simulink model "ABS_Regen_Straight"  (R2023a)
settings: Solver=ode45  StartTime=0  StopTime=15  FixedStep=0.002  RelTol=1e-3  AbsTol=1e-6
libraries: Solver_SF x1, cstblocks x1
settings Model: ExtModeTrigMode=oneshot  VariantFading=off  Creator=ywata  LastModifiedBy=USER
settings SolverCC: AutoScaleAbsTol=off  AlgebraicLoopSolver=TrustRegion
settings DataIOCC: SaveFormat=Array  SignalLoggingSaveFormat=ModelDataLogs  ReturnWorkspaceOutputs=off  SignalLoggingName=sigsOut
settings OptimizationCC: BlockReduction=off  BooleanDataType=off  ExpressionDepthLimit=2147483647  LifeSpan=inf
settings DebuggingCC: SaveWithParameterizedLinksMsg=none  UnderspecifiedInitializationDetection=Classic  MergeDetectMultiDrivingBlocksExec=none  SignalResolutionControl=TryResolveAllWithWarning  MultiTaskDSMMsg=warning  MultiTaskCondExecSysMsg=none  FcnCallInpInsideContextMsg=warning  UnconnectedInputMsg=warning  UnconnectedOutputMsg=warning  UnconnectedLineMsg=warning  StateNameClashWarn=warning  SFUnexpectedBacktrackingDiag=warning  SFNoUnconditionalDefaultTransitionDiag=warning  SFExecutionAtInitializationDiag=none  ArithmeticOperatorsInVariantConditions=warning
settings HardwareCC: ProdBitPerPointer=32  ProdBitPerSizeT=32  ProdBitPerPtrDiffT=32  ProdLargestAtomicFloat=None  ProdIntDivRoundTo=Undefined  ProdEndianess=Unspecified  ProdWordSize=32  ProdHWDeviceType=32-bit Generic  TargetUnknown=on
settings ModelReferenceCC: PropagateSignalLabelsOutOfModel=off
settings SFSimCC: SimUseLocalCustomCode=off  CustomCodeUndefinedFunction=UseInterfaceOnly
settings RTWCC: TemplateMakefile=grt_vc.tmf  RTWUseLocalCustomCode=off
settings CodeAppCC: StateflowObjectComments=on
settings GRTTargetCC: TargetFcnLib=ansi_tfl_tmw.mat  TargetLangStandard=C89/C90 (ANSI)  CombineOutputUpdateFcns=off  GRTInterface=on
settings ConfigComp: CovMetricSettings=dw  CovSaveCumulativeToWorkspaceVar=on  CovSaveSingleToWorkspaceVar=on  CovExternalEMLEnable=off

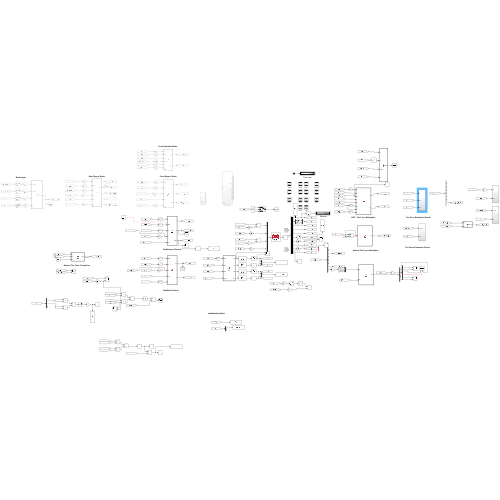
[thumbnail: Simulink's stored preview of the top-level diagram]
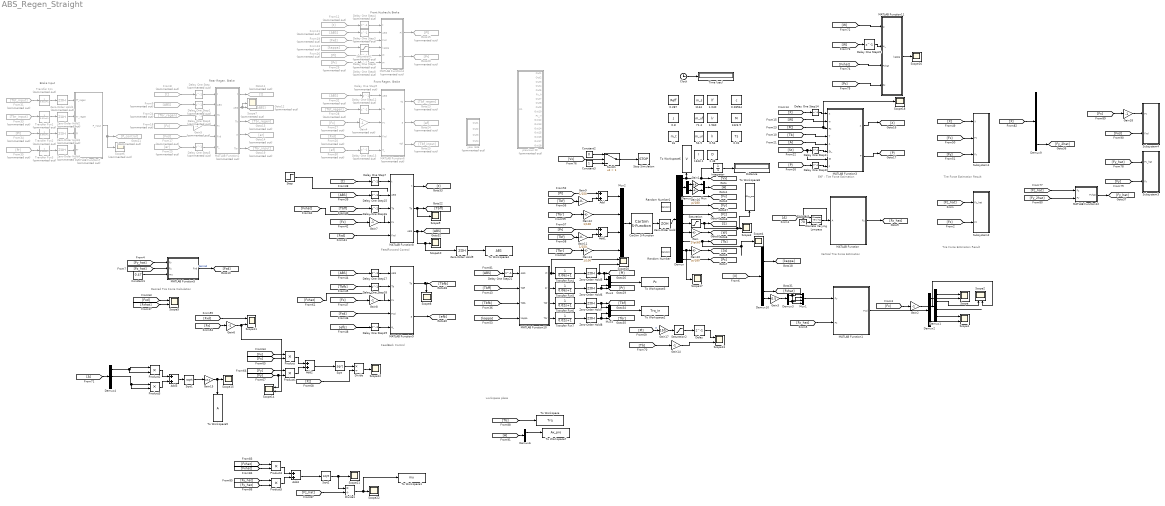
== system ABS_Regen_Straight ==
  note: workspace place
  note: Front Hydraulic Brake
  note: EKF : Tire Force Estimation
  note: Tire Force Estimation Result
  note: Vertical Tire Force Estimation
  note: Tire Force Estimation Result
  note: Rear Regen. Brake
  note: Desired Tire Force Calculation
  note: Front Regen. Brake
  note: Brake Input
  note: FeedForward Control
  note: FeedBack Control
  0.01 : DataStoreMemory  DataStoreName=Ts  WriteAfterWriteMsg=warning  InitialValue=0.01  ShowAdditionalParam=off  OutDataTypeStr=double
  0.287 : DataStoreMemory  DataStoreName=Reff  WriteAfterWriteMsg=warning  InitialValue=0.287  ShowAdditionalParam=off  OutDataTypeStr=double
  0.28944 : DataStoreMemory  DataStoreName=c  WriteAfterWriteMsg=warning  InitialValue=0.29844  ShowAdditionalParam=off  OutDataTypeStr=double
  0.54 : DataStoreMemory  DataStoreName=h  WriteAfterWriteMsg=warning  InitialValue=0.54  ShowAdditionalParam=off  OutDataTypeStr=double
  0.8 : DataStoreMemory  DataStoreName=J  WriteAfterWriteMsg=warning  InitialValue=0.8  ShowAdditionalParam=off  OutDataTypeStr=double
  1.040 : DataStoreMemory  DataStoreName=lf  WriteAfterWriteMsg=warning  InitialValue=1.040  ShowAdditionalParam=off  OutDataTypeStr=double
  1.48 : DataStoreMemory  DataStoreName=D  WriteAfterWriteMsg=warning  InitialValue=1.48  ShowAdditionalParam=off  OutDataTypeStr=double
  1.560 : DataStoreMemory  DataStoreName=lr  WriteAfterWriteMsg=warning  InitialValue=1.560  ShowAdditionalParam=off  OutDataTypeStr=double
  1134 : DataStoreMemory  DataStoreName=m_s  WriteAfterWriteMsg=warning  InitialValue=1134  ShowAdditionalParam=off  OutDataTypeStr=double
  1323.9 : DataStoreMemory  DataStoreName=M  WriteAfterWriteMsg=warning  InitialValue=1323.9  ShowAdditionalParam=off  OutDataTypeStr=double
  1343.1 : DataStoreMemory  DataStoreName=I  WriteAfterWriteMsg=warning  InitialValue=1343.1  ShowAdditionalParam=off  OutDataTypeStr=double
  16 : DataStoreMemory  DataStoreName=m_t  WriteAfterWriteMsg=warning  InitialValue=16  ShowAdditionalParam=off  OutDataTypeStr=double
  54.5 : DataStoreMemory  DataStoreName=m_ur  WriteAfterWriteMsg=warning  InitialValue=54.5  ShowAdditionalParam=off  OutDataTypeStr=double
  71.4 : DataStoreMemory  DataStoreName=m_uf  WriteAfterWriteMsg=warning  InitialValue=71.4  ShowAdditionalParam=off  OutDataTypeStr=double
  Add{,1..4} (5 alike) : Sum
  CarSim S-Function : Solver_SF/CarSim S-Function  Priority=1  SIMFILE=simfile.sim  Run_RTs=off  vs_state_ind=Run  StopMode_ind=Vehicle Model
  Clock : Clock
  Constant : Constant  Value=70  SampleTime=0.01
  Constant1 : Constant  Value=0.47
  Constant2 : Constant  Value=0
  Constant3 : Constant
  Delay : Delay  DelayLength=1
  Delay One Step : Delay  Commented=on  DelayLength=1  InitialCondition=-0.01
  Delay One Step{1,3,5..6,8..9,13} (7 alike) : Delay  Commented=on  DelayLength=1  InitialCondition=0
  Delay One Step10 : Delay  DelayLength=1  InitialCondition=diag([67.655 67.655 67.655 67.655 10 0 0 0 0 0 0 0 0 0 0 0])
  Delay One Step11 : Delay  DelayLength=1  InitialCondition=[0 0]'
  Delay One Step12 : Delay  Commented=on  DelayLength=1  InitialCondition=[0 0 0 0]'
  Delay One Step14 : Delay  DelayLength=1  InitialCondition=[67.655 67.655 67.655 67.655 10 0 0 0 0 0 0 0 0 0 0 0]'
  Delay One Step15 : Delay  DelayLength=1  InitialCondition=0
  Delay One Step16 : Delay  DelayLength=1  InitialCondition=[0 0 0 0]'
  Delay One Step17 : Delay  DelayLength=1  InitialCondition=0
  Delay One Step18 : Delay  DelayLength=1  InitialCondition=[0 0 0 0]'
  Delay One Step19 : Delay  DelayLength=1  InitialCondition=[0 0 0 0]'
  Delay One Step2 : Delay  Commented=on  DelayLength=1  InitialCondition=[0 0 0 0]'
  Delay One Step20 : Delay  DelayLength=1  InitialCondition=[67.655,67.655,67.655,67.655]'
  Delay One Step21 : Delay  DelayLength=1  InitialCondition=0
  Delay One Step4 : Delay  Commented=on  DelayLength=1  InitialCondition=-0.01
  Delay One Step7 : Delay  DelayLength=1  InitialCondition=-0.01
  Demux : Demux  Outputs=[1 3 4 4 4 4 4 4 2 2]
  Demux1 : Demux
  Demux10 : Demux  Outputs=[4 1 2 1 2 4 2]
  Demux2 : Demux
  Demux3 : Demux  Outputs=2
  Demux4 : Demux  Outputs=3
  Demux5 : Demux  Outputs=[2 1]
  Demux6 : Demux  Outputs=3
  Demux9 : Demux  Outputs=[4 1 2 1 2 4 2]
  Discrete Varying Lowpass : cstblocks/Linear Parameter Varying/Discrete Varying Lowpass  N=1  w0=0  Ts=0.01
  Distance : Display
      settings: Format=bank  Decimation=100
  Divide : Product  Inputs=*/
  Divide1 : Product  Inputs=*/
  From{1,21,71,91} (4 alike) : From
  From11 : From  Commented=on  GotoTag=ABS
  From12 : From  Commented=on  GotoTag=t
  From13 : From  Commented=on  GotoTag=kappa
  From17 : From  Commented=on  GotoTag=Fxd
  From18 : From  Commented=on  GotoTag=Fx
  From19 : From  Commented=on  GotoTag=Fxd
  From20 : From  Commented=on  GotoTag=Fxd
  From24 : From  Commented=on  GotoTag=Tbr_regen
  From25 : From  Commented=on  GotoTag=er
  From26 : From  Commented=on  GotoTag=Pl
  From27 : From  Commented=on  GotoTag=Fx
  From28 : From  Commented=on  GotoTag=Tbf_regen
  From29 : From  Commented=on  GotoTag=Pr
  From30 : From  Commented=on  GotoTag=ef
  From31 : From  Commented=on  GotoTag=Tbf_input
  From32 : From  Commented=on  GotoTag=ABS
  From33 : From  Commented=on  GotoTag=Tbr_input
  From34 : From  Commented=on  GotoTag=Pl
  From35 : From  Commented=on  GotoTag=Pr
  From8 : From  Commented=on  GotoTag=t
  From9 : From  Commented=on  GotoTag=ABS
  Gain : Gain  Gain=2*pi/60
  Gain1 : Gain  Gain=9.8
  Gain10 : Gain  Gain=pi/180
  Gain11 : Gain  Gain=1/150
  Gain12 : Gain  Gain=1/100
  Gain13 : Gain  Gain=1/100
  Gain{2,6..8,14,18} (6 alike) : Gain  Gain=-1
  Gain15 : Gain  Gain=1/9.8
  Gain16 : Gain  Gain=pi/180
  Gain17 : Gain  Gain=150
  Gain3 : Gain  Gain=0.5
  Gain4 : Gain  Commented=on  Gain=-1
  Gain5 : Gain  Commented=on  Gain=-1
  Gain9 : Gain  Gain=1/150
  Goto1 : Goto
  Goto11 : Goto  Commented=on  GotoTag=t
  Goto12 : Goto  Commented=on  GotoTag=ABS
  Goto13 : Goto  Commented=on  GotoTag=Tbr_regen
  Goto14 : Goto  Commented=on  GotoTag=er
  Goto15 : Goto  Commented=on  GotoTag=Pl
  Goto19 : Goto  Commented=on  GotoTag=Tbr_input
  Goto20 : Goto  Commented=on  GotoTag=Pr
  Goto21 : Goto  Commented=on  GotoTag=P_control
  Goto23 : Goto  Commented=on  GotoTag=Tbf_regen
  Goto24 : Goto  Commented=on  GotoTag=ef
  Goto25 : Goto  Commented=on  GotoTag=Tbf_input
  Integrator : Integrator
  MATLAB Function : MATLAB Function  TreatAsAtomicUnit=on
  MATLAB Function1 : MATLAB Function  TreatAsAtomicUnit=on
  MATLAB Function10 : MATLAB Function  TreatAsAtomicUnit=on
  MATLAB Function11 : MATLAB Function  TreatAsAtomicUnit=on
  MATLAB Function12 : MATLAB Function  TreatAsAtomicUnit=on
  MATLAB Function2 : MATLAB Function  Commented=on  TreatAsAtomicUnit=on
  MATLAB Function3 : MATLAB Function  TreatAsAtomicUnit=on
  MATLAB Function4 : MATLAB Function  Commented=on  TreatAsAtomicUnit=on
  MATLAB Function5 : MATLAB Function  TreatAsAtomicUnit=on
  MATLAB Function6 : MATLAB Function  Commented=on  TreatAsAtomicUnit=on
  MATLAB Function7 : MATLAB Function  Commented=on  TreatAsAtomicUnit=on
  MATLAB Function8 : MATLAB Function  TreatAsAtomicUnit=on
  MATLAB Function9 : MATLAB Function  TreatAsAtomicUnit=on
  Mux : Mux  Inputs=2
  Mux1 : Mux
  Mux2 : Mux
  Mux3 : Mux  Inputs=2
  Mux4 : Mux  Inputs=2
  Product{,1..5} (6 alike) : Product
  Random Number : RandomNumber  Variance=0.01^2  SampleTime=0.01
  Random Number1 : RandomNumber  Variance=0.01  SampleTime=0.01
  Saturation : Saturate  UpperLimit=1  LowerLimit=-1
  Saturation1 : Saturate  Commented=on  UpperLimit=200  LowerLimit=100
  Saturation2 : Saturate  UpperLimit=1000  LowerLimit=0
  Scope{,1..2,5,11,13..14,20} (8 alike) : Scope  NumInputPorts=2
  Scope{3..4,8..10,12,15..18,21..22} (12 alike) : Scope
  Scope6 : Scope  Commented=on
  Scope7 : Scope  Commented=on
  Sqrt : Sqrt
  Sqrt1 : Sqrt
  Sqrt2 : Sqrt
  Step : Step  Time=5.34  SampleTime=0.01
  Stop Simulation : Stop
  Subsystem1 : Subsystem
  Subsystem2 : Subsystem
  Subsystem3 : Subsystem
  Subsystem4 : Subsystem
  Switch : Switch  Criteria=u2 > Threshold  Threshold=1  SaturateOnIntegerOverflow=off  InputSameDT=off
  Time (sec) : Display
      settings: Format=bank  Decimation=100
  To Workspace : ToWorkspace  VariableName=Trq  SaveFormat=Timeseries  SampleTime=-1
  To Workspace1 : ToWorkspace  VariableName=mu  SaveFormat=Timeseries  SampleTime=-1
  To Workspace2 : ToWorkspace  VariableName=Trq_in  SaveFormat=Timeseries  SampleTime=-1
  To Workspace3 : ToWorkspace  VariableName=Pc  SaveFormat=Timeseries  SampleTime=-1
  To Workspace4 : ToWorkspace  VariableName=ABS  SaveFormat=Timeseries  SampleTime=-1
  To Workspace5 : ToWorkspace  VariableName=A  SaveFormat=Timeseries  SampleTime=-1
  To Workspace6 : ToWorkspace  VariableName=V  SaveFormat=Timeseries  SampleTime=-1
  To Workspace7 : ToWorkspace  VariableName=Ax_pro  SaveFormat=Timeseries  SampleTime=-1
  To Workspace8 : ToWorkspace  VariableName=Slip_pro  SaveFormat=Timeseries  SampleTime=-1
  Transfer Fcn : TransferFcn  Commented=on  Denominator=[0.02 1]
  Transfer Fcn1 : TransferFcn  Commented=on  Denominator=[0.02 1]
  Transfer Fcn2 : TransferFcn  Commented=on  Denominator=[0.06 1]
  Transfer Fcn3 : TransferFcn  Commented=on  Denominator=[0.06 1]
  Transfer Fcn4 : TransferFcn  Denominator=[0.06 1]
  Transfer Fcn5 : TransferFcn  Denominator=[0.06 1]
  Transfer Fcn6 : TransferFcn  Denominator=[0.02 1]
  Transfer Fcn7 : TransferFcn  Denominator=[0.02 1]
  Zero-Order Hold{,5..9} (6 alike) : ZeroOrderHold  SampleTime=0.01
  Zero-Order Hold{1..4} (4 alike) : ZeroOrderHold  Commented=on  SampleTime=0.01
  previous KF : Subsystem  Commented=on
  yaw rate : Subsystem  Commented=on
  wires:
  CarSim S-Function/1 -> Zero-Order Hold/1
  Clock/1 -> Time (sec)/1
  Demux/1 -> Integrator/1, [Vx], To Workspace6/1
  Demux/3 -> [Fx]
  Zero-Order Hold/1 -> Demux/1
  Saturation/1 -> To Workspace8/1, Scope3/1, [S]
  Gain/1 -> [W]
  Demux/2 -> Demux5/1
  Demux5/1 -> Gain1/1
  Mux/1 -> Goto1/1
  Demux5/2 -> Gain16/1
  Gain1/1 -> Mux/1
  Demux/10 -> [Pc]
  Demux/9 -> Scope17/1, Gain10/1
  Demux/8 -> Scope4/1, [Tb]
  Demux/7 -> Gain/1
  Demux/6 -> Saturation/1
  Demux/5 -> [Fz]
  Demux/4 -> [Fy]
  Gain16/1 -> Mux/2
  Delay One Step11/1 -> MATLAB Function3/6(St_)
  From21/1 -> MATLAB Function3/5(A)
  [P] -> Delay One Step10/1
  [Tb] -> MATLAB Function3/4(T)
  [W] -> MATLAB Function3/2(w)
  [X] -> Delay One Step14/1
  [St] -> MATLAB Function3/7(St), Delay One Step11/1
  MATLAB Function3/2(P) -> [P]
  Delay One Step10/1 -> MATLAB Function3/8("P ")
  MATLAB Function3/1(X) -> [X]
  [Pc] -> Scope18/1, MATLAB Function3/3(Pc)
  Delay One Step14/1 -> MATLAB Function3/1("X ")
  Gain10/1 -> [St]
  [X] -> Subsystem1/1(X)
  [Fx] -> Subsystem1/2(Fx)
  [Fy] -> Subsystem1/3(Fy)
  From1/1 -> MATLAB Function/1(A), Discrete Varying Lowpass/1
  MATLAB Function/1(Fz) -> [Fz_hat]
  [Fz_hat] -> Subsystem2/1(Fz_hat)
  [Fz] -> Subsystem2/2(Fz)
  Constant/1 -> Discrete Varying Lowpass/2
  Discrete Varying Lowpass/1 -> ?
  [Fz_hat] -> MATLAB Function1/2(Fz)
  MATLAB Function1/1(Fxd) -> Demux2/1
  [Fx] -> Gain2/1
  Gain2/1 -> Demux1/1
  Demux1/1 -> Scope/1
  Demux2/1 -> Scope/2
  Demux1/4 -> Scope1/1
  Demux2/4 -> Scope1/2
  [X] -> Demux10/1
  Demux10/7 -> Gain3/1
  Gain3/1 -> Demux3/1
  Demux3/1 -> Mux1/3, Mux1/1
  Mux1/1 -> MATLAB Function1/1(Fy)
  Demux3/2 -> Mux1/4, Mux1/2
  Demux1/2 -> Scope2/1
  Demux1/3 -> ?
  MATLAB Function2/1(t) -> Goto11/1
  MATLAB Function2/2(ABS) -> Scope7/1, Goto12/1
  [Fy_hat] -> MATLAB Function5/1(Fy)
  [Fz_hat] -> MATLAB Function5/2(Fz)
  MATLAB Function5/1(Fxd) -> [Fxd]  "desired"
  From8/1 -> Delay One Step/1
  Delay One Step/1 -> MATLAB Function2/1("t ")
  From9/1 -> Delay One Step1/1
  Delay One Step1/1 -> MATLAB Function2/2("ABS ")
  From11/1 -> Delay One Step3/1
  Delay One Step3/1 -> MATLAB Function4/2(ABS)
  From12/1 -> Delay One Step4/1
  Delay One Step4/1 -> MATLAB Function4/1(t)
  From17/1 -> MATLAB Function2/5(Fxd)
  From18/1 -> Gain5/1
  Gain5/1 -> MATLAB Function2/4(Fx)
  From19/1 -> MATLAB Function4/3(Fxd)
  MATLAB Function2/3(Tb) -> Goto13/1
  From24/1 -> Delay One Step2/1
  Delay One Step2/1 -> MATLAB Function2/3("Tb ")
  MATLAB Function2/4(e) -> Goto14/1
  From25/1 -> Delay One Step5/1
  Delay One Step5/1 -> MATLAB Function2/6(e_)
  Demux10/2 -> [kappa]
  From13/1 -> Saturation1/1
  MATLAB Function2/5(Tbr) -> Goto19/1
  MATLAB Function4/1(Pl) -> Goto15/1
  MATLAB Function4/2(Pr) -> Goto20/1
  From26/1 -> Delay One Step6/1
  Delay One Step6/1 -> MATLAB Function4/5("Pl ")
  Delay One Step8/1 -> MATLAB Function4/6("Pr ")
  From29/1 -> Delay One Step8/1
  Saturation1/1 -> MATLAB Function4/4(kappa)
  From30/1 -> Delay One Step13/1
  From28/1 -> Delay One Step12/1
  Delay One Step12/1 -> MATLAB Function6/2("Tb ")
  Delay One Step13/1 -> MATLAB Function6/5(e_)
  MATLAB Function6/1(Tb) -> Goto23/1
  From27/1 -> Gain4/1
  Delay One Step9/1 -> MATLAB Function6/1(ABS)
  MATLAB Function6/2(e) -> Goto24/1
  Gain4/1 -> MATLAB Function6/3(Fx)
  MATLAB Function6/3(Tbf) -> Goto25/1
  From32/1 -> Delay One Step9/1
  From20/1 -> MATLAB Function6/4(Fxd)
  From31/1 -> Transfer Fcn/1
  From33/1 -> Transfer Fcn1/1
  From34/1 -> Transfer Fcn2/1
  From35/1 -> Transfer Fcn3/1
  MATLAB Function7/1(P_input) -> Scope6/1, Goto21/1
  Transfer Fcn/1 -> Zero-Order Hold1/1
  Transfer Fcn1/1 -> Zero-Order Hold2/1
  Transfer Fcn2/1 -> Zero-Order Hold3/1
  Transfer Fcn3/1 -> Zero-Order Hold4/1
  Zero-Order Hold1/1 -> MATLAB Function7/1(Tf_regen)
  Zero-Order Hold2/1 -> MATLAB Function7/2(Tr_regen)
  Zero-Order Hold3/1 -> MATLAB Function7/3(Pl)
  Zero-Order Hold4/1 -> MATLAB Function7/4(Pr)
  Constant1/1 -> MATLAB Function5/3(mu)
  [ABS] -> Delay One Step15/1
  Delay One Step7/1 -> MATLAB Function8/1("t ")
  [t] -> Delay One Step7/1
  Delay One Step15/1 -> MATLAB Function8/2("ABS ")
  MATLAB Function8/2(Tb) -> Scope9/1, [Tbff]
  [Tbff] -> Delay One Step16/1
  Delay One Step16/1 -> MATLAB Function8/3("Tb ")
  Gain7/1 -> ?
  [Fxd] -> MATLAB Function8/5(Fxd)
  [Fx] -> Gain7/1
  [Fxd] -> MATLAB Function9/4(Fxd)
  Delay One Step18/1 -> MATLAB Function9/2("Tb ")
  [Fx] -> Gain8/1
  [Tbfb] -> Delay One Step18/1
  Gain8/1 -> ?
  Delay One Step17/1 -> MATLAB Function9/1(ABS)
  [ABS] -> Delay One Step17/1
  MATLAB Function9/2(e) -> [efb]
  MATLAB Function9/1(Tb) -> Scope8/1, [Tbfb]
  [efb] -> Delay One Step19/1
  Delay One Step19/1 -> MATLAB Function9/5(e_)
  Demux10/6 -> [Fxhat]
  MATLAB Function8/3(ABS) -> Zero-Order Hold9/1, Scope10/1, [ABS]
  MATLAB Function8/1(t) -> [t]
  [Fxd] -> Scope11/1
  [Fx] -> Gain6/1
  [Tbfb] -> MATLAB Function10/3(Tbfb)
  [Tbff] -> MATLAB Function10/2(Tbff)
  [kappa] -> MATLAB Function10/4(kappa)
  MATLAB Function10/1(Pl) -> Scope20/1, Transfer Fcn4/1
  Add/1 -> Mux2/1
  [Pl] -> Add/1
  [Tbf] -> Gain9/1
  Gain9/1 -> Add/2
  [Tbf] -> Gain11/1
  Add1/1 -> Mux2/3
  [Pr] -> Add1/1
  Gain11/1 -> Add1/2
  MATLAB Function10/2(Pr) -> Transfer Fcn5/1
  MATLAB Function10/3(Tbf) -> Transfer Fcn6/1
  MATLAB Function10/4(Tbr) -> Transfer Fcn7/1
  [Tbr] -> Gain12/1
  Gain12/1 -> Mux2/2
  Gain13/1 -> Mux2/4
  [Tbr] -> Gain13/1
  [Fxhat] -> MATLAB Function9/3(Fx)
  [Fxhat] -> MATLAB Function8/4(Fx)
  [Fxd] -> Scope5/1
  Gain6/1 -> Scope11/2, Scope14/2
  [Fxhat] -> Scope5/2
  Transfer Fcn4/1 -> Zero-Order Hold5/1
  Transfer Fcn5/1 -> Zero-Order Hold6/1
  Transfer Fcn6/1 -> Zero-Order Hold7/1
  Transfer Fcn7/1 -> Zero-Order Hold8/1
  Zero-Order Hold5/1 -> Scope20/2, Mux3/1, [Pl]
  Zero-Order Hold6/1 -> Mux3/2, [Pr]
  Zero-Order Hold7/1 -> Mux4/1, [Tbf]
  Zero-Order Hold8/1 -> Mux4/2, [Tbr]
  [Fx] -> Product/1
  [Fx] -> Product/2
  [Fy] -> Scope14/1, Product1/2
  [Fy] -> Product1/1
  Product/1 -> Add2/1
  Product1/1 -> Add2/2
  Add2/1 -> Sqrt/1
  Sqrt/1 -> Divide/1
  [Fz] -> Divide/2
  Divide/1 -> Scope12/1
  [Pl] -> Gain17/1  "in"
  [Tb] -> Gain14/1
  Gain14/1 -> Scope13/2
  Saturation2/1 -> Delay/1
  Delay/1 -> Scope13/1
  From71/1 -> Demux4/1
  Product3/1 -> Add3/2
  Product2/1 -> Add3/1
  Add3/1 -> Sqrt1/1
  Demux4/1 -> Product2/2, Product2/1
  Demux4/2 -> Product3/2, Product3/1
  Sqrt1/1 -> Gain15/1
  Gain15/1 -> To Workspace5/1, Scope15/1
  Demux2/2 -> Scope2/2
  [W] -> MATLAB Function11/1(w)
  [W] -> Delay One Step20/1
  Delay One Step20/1 -> MATLAB Function11/2(w_)
  [Pc] -> MATLAB Function11/4(Pc)
  [Fxhat] -> MATLAB Function11/3(Fxhat)
  MATLAB Function11/1(kappa) -> Scope16/1
  [Vx] -> Switch/2
  Constant2/1 -> Switch/1
  Constant3/1 -> Switch/3
  Switch/1 -> Stop Simulation/1
  [X] -> Demux9/1
  Demux9/7 -> [Fy_2hat]
  [Fz_hat] -> MATLAB Function12/1(Fz)
  [Fy_2hat] -> MATLAB Function12/2(Fy)
  MATLAB Function12/1(Fyhat) -> [Fy_hat]
  [Fy] -> Subsystem3/2(Fy)
  [Fy_hat] -> Subsystem3/1(Fy_hat)
  Gain17/1 -> Saturation2/1
  [ABS] -> Delay One Step21/1
  Delay One Step21/1 -> MATLAB Function10/1(ABS)
  Product4/1 -> Add4/1
  [Fy_hat] -> Product5/2
  [Fy_hat] -> Product5/1
  [Fxhat] -> Product4/2
  Add4/1 -> Sqrt2/1
  [Fxhat] -> Product4/1
  Product5/1 -> Add4/2
  Sqrt2/1 -> Divide1/1, Scope21/1
  [Fz_hat] -> Divide1/2
  Divide1/1 -> To Workspace1/1, Scope22/1
  [Tb] -> To Workspace/1
  Mux3/1 -> To Workspace3/1
  Mux4/1 -> To Workspace2/1
  Zero-Order Hold9/1 -> To Workspace4/1
  [Fxd] -> Subsystem4/2(Fxd)
  [Fx] -> Gain18/1
  From91/1 -> Demux6/1
  Demux6/1 -> To Workspace7/1
  Integrator/1 -> Distance/1
  Gain18/1 -> Subsystem4/1(Fx)
  Step/1 -> ?
  Mux2/1 -> CarSim S-Function/1

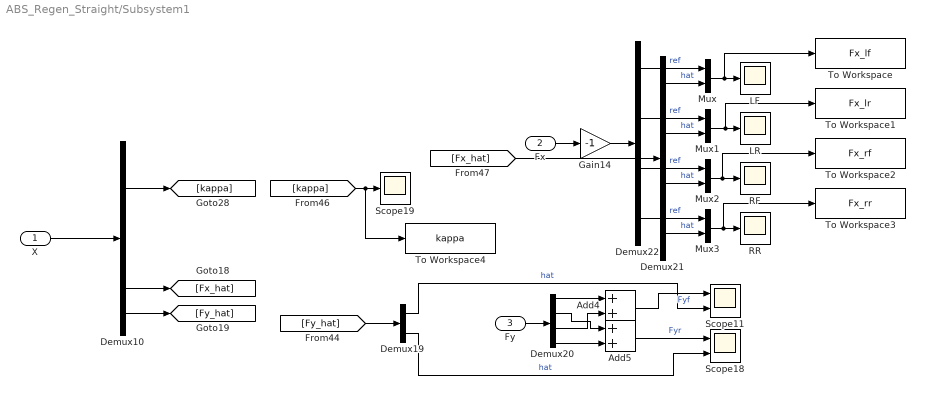
== system ABS_Regen_Straight/Subsystem1 ==
  X : Inport
  Fx : Inport  Port=2
  Fy : Inport  Port=3
  Add4 : Sum
  Add5 : Sum
  Demux10 : Demux  Outputs=[4 1 2 1 2 4 2]
  Demux19 : Demux  Outputs=2
  Demux20 : Demux
  Demux21 : Demux
  Demux22 : Demux
  Gain14 : Gain  Gain=-1
  LF : Scope
  LR : Scope
  Mux{,1..3} (4 alike) : Mux  Inputs=2
  RF : Scope
  RR : Scope
  Scope11 : Scope  NumInputPorts=2
  Scope18 : Scope  NumInputPorts=2
  Scope19 : Scope
  To Workspace : ToWorkspace  VariableName=Fx_lf  SaveFormat=Timeseries  SampleTime=-1
  To Workspace1 : ToWorkspace  VariableName=Fx_lr  SaveFormat=Timeseries  SampleTime=-1
  To Workspace2 : ToWorkspace  VariableName=Fx_rf  SaveFormat=Timeseries  SampleTime=-1
  To Workspace3 : ToWorkspace  VariableName=Fx_rr  SaveFormat=Timeseries  SampleTime=-1
  To Workspace4 : ToWorkspace  VariableName=kappa  SaveFormat=Timeseries  SampleTime=-1
  wires:
  Demux21/3 -> Mux2/2  "hat"
  [Fx_hat] -> Demux21/1
  Add5/1 -> Scope18/1  "Fyr"
  [Fy_hat] -> Demux19/1
  Demux21/4 -> Mux3/2  "hat"
  Fx/1 -> Gain14/1
  Gain14/1 -> Demux22/1
  Demux22/4 -> Mux3/1  "ref"
  Demux20/1 -> Add4/1
  Demux10/2 -> [kappa]
  Demux19/1 -> Scope11/2  "hat"
  Demux19/2 -> Scope18/2  "hat"
  Demux21/1 -> Mux/2  "hat"
  Demux20/2 -> Add5/1
  Demux22/3 -> Mux2/1  "ref"
  Demux20/4 -> Add5/2
  Demux20/3 -> Add4/2
  Demux10/7 -> [Fy_hat]
  Fy/1 -> Demux20/1
  Demux22/2 -> Mux1/1  "ref"
  Demux21/2 -> Mux1/2  "hat"
  X/1 -> Demux10/1
  Add4/1 -> Scope11/1  "Fyf"
  Demux10/6 -> [Fx_hat]
  [kappa] -> To Workspace4/1, Scope19/1
  Demux22/1 -> Mux/1  "ref"
  Mux/1 -> To Workspace/1, LF/1
  Mux1/1 -> To Workspace1/1, LR/1
  Mux2/1 -> To Workspace2/1, RF/1
  Mux3/1 -> To Workspace3/1, RR/1

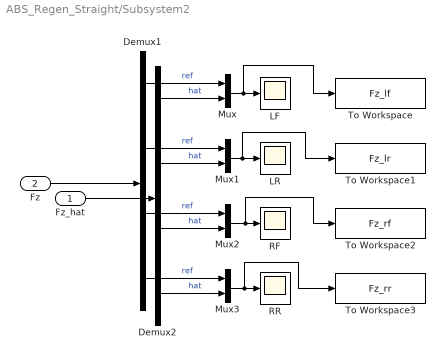
== system ABS_Regen_Straight/Subsystem2 ==
  Fz_hat : Inport
  Fz : Inport  Port=2
  Demux1 : Demux
  Demux2 : Demux
  LF : Scope
  LR : Scope
  Mux{,1..3} (4 alike) : Mux  Inputs=2
  RF : Scope
  RR : Scope
  To Workspace : ToWorkspace  VariableName=Fz_lf  SaveFormat=Timeseries  SampleTime=-1
  To Workspace1 : ToWorkspace  VariableName=Fz_lr  SaveFormat=Timeseries  SampleTime=-1
  To Workspace2 : ToWorkspace  VariableName=Fz_rf  SaveFormat=Timeseries  SampleTime=-1
  To Workspace3 : ToWorkspace  VariableName=Fz_rr  SaveFormat=Timeseries  SampleTime=-1
  wires:
  Fz_hat/1 -> Demux2/1
  Fz/1 -> Demux1/1
  Demux1/1 -> Mux/1  "ref"
  Demux2/1 -> Mux/2  "hat"
  Demux2/2 -> Mux1/2  "hat"
  Demux1/2 -> Mux1/1  "ref"
  Demux1/3 -> Mux2/1  "ref"
  Demux2/3 -> Mux2/2  "hat"
  Demux1/4 -> Mux3/1  "ref"
  Demux2/4 -> Mux3/2  "hat"
  Mux/1 -> To Workspace/1, LF/1
  Mux1/1 -> To Workspace1/1, LR/1
  Mux2/1 -> To Workspace2/1, RF/1
  Mux3/1 -> To Workspace3/1, RR/1

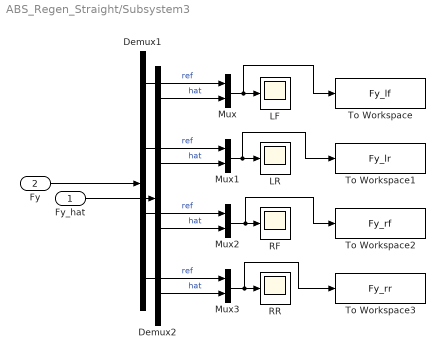
== system ABS_Regen_Straight/Subsystem3 ==
  Fy_hat : Inport
  Fy : Inport  Port=2
  Demux1 : Demux
  Demux2 : Demux
  LF : Scope
  LR : Scope
  Mux{,1..3} (4 alike) : Mux  Inputs=2
  RF : Scope
  RR : Scope
  To Workspace : ToWorkspace  VariableName=Fy_lf  SaveFormat=Timeseries  SampleTime=-1
  To Workspace1 : ToWorkspace  VariableName=Fy_lr  SaveFormat=Timeseries  SampleTime=-1
  To Workspace2 : ToWorkspace  VariableName=Fy_rf  SaveFormat=Timeseries  SampleTime=-1
  To Workspace3 : ToWorkspace  VariableName=Fy_rr  SaveFormat=Timeseries  SampleTime=-1
  wires:
  Fy_hat/1 -> Demux2/1
  Fy/1 -> Demux1/1
  Demux1/1 -> Mux/1  "ref"
  Demux2/1 -> Mux/2  "hat"
  Demux2/2 -> Mux1/2  "hat"
  Demux1/2 -> Mux1/1  "ref"
  Demux1/3 -> Mux2/1  "ref"
  Demux2/3 -> Mux2/2  "hat"
  Demux1/4 -> Mux3/1  "ref"
  Demux2/4 -> Mux3/2  "hat"
  Mux/1 -> To Workspace/1, LF/1
  Mux1/1 -> To Workspace1/1, LR/1
  Mux2/1 -> To Workspace2/1, RF/1
  Mux3/1 -> To Workspace3/1, RR/1

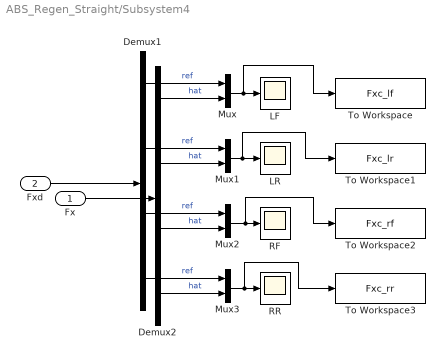
== system ABS_Regen_Straight/Subsystem4 ==
  Fx : Inport
  Fxd : Inport  Port=2
  Demux1 : Demux
  Demux2 : Demux
  LF : Scope
  LR : Scope
  Mux{,1..3} (4 alike) : Mux  Inputs=2
  RF : Scope
  RR : Scope
  To Workspace : ToWorkspace  VariableName=Fxc_lf  SaveFormat=Timeseries  SampleTime=-1
  To Workspace1 : ToWorkspace  VariableName=Fxc_lr  SaveFormat=Timeseries  SampleTime=-1
  To Workspace2 : ToWorkspace  VariableName=Fxc_rf  SaveFormat=Timeseries  SampleTime=-1
  To Workspace3 : ToWorkspace  VariableName=Fxc_rr  SaveFormat=Timeseries  SampleTime=-1
  wires:
  Fx/1 -> Demux2/1
  Fxd/1 -> Demux1/1
  Demux1/1 -> Mux/1  "ref"
  Demux2/1 -> Mux/2  "hat"
  Demux2/2 -> Mux1/2  "hat"
  Demux1/2 -> Mux1/1  "ref"
  Demux1/3 -> Mux2/1  "ref"
  Demux2/3 -> Mux2/2  "hat"
  Demux1/4 -> Mux3/1  "ref"
  Demux2/4 -> Mux3/2  "hat"
  Mux/1 -> To Workspace/1, LF/1
  Mux1/1 -> To Workspace1/1, LR/1
  Mux2/1 -> To Workspace2/1, RF/1
  Mux3/1 -> To Workspace3/1, RR/1

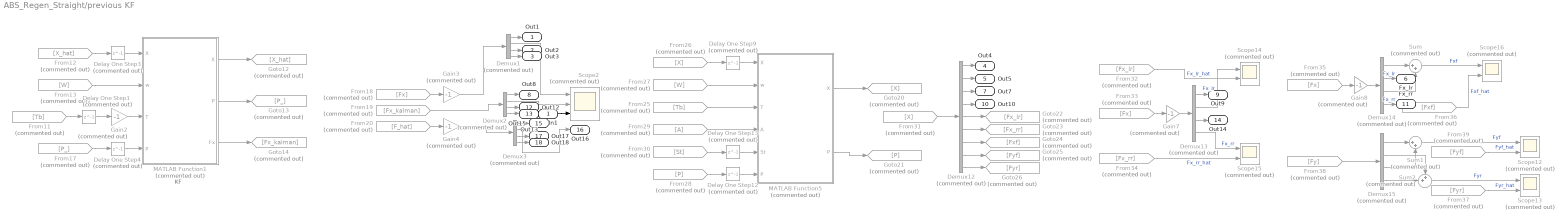
== system ABS_Regen_Straight/previous KF ==
  note: KF
  In1 : Inport
  Delay One Step1 : Delay  Commented=on  DelayLength=1  InitialCondition=zeros(4,1)
  Delay One Step12 : Delay  Commented=on  DelayLength=1  InitialCondition=diag([67.655 67.655 0 0 0 0 0 0 0])
  Delay One Step13 : Delay  Commented=on  DelayLength=1  InitialCondition=[0 0]'
  Delay One Step3 : Delay  Commented=on  DelayLength=1  InitialCondition=[67.655 67.655 67.655 67.655; 0 0 0 0]
  Delay One Step4 : Delay  Commented=on  DelayLength=1  InitialCondition=10*ones(2,8)
  Delay One Step9 : Delay  Commented=on  DelayLength=1  InitialCondition=[67.655 67.655 0 0 0 0 0 0 0]'
  Demux{1..3,13..15} (6 alike) : Demux  Commented=on
  Demux12 : Demux  Commented=on  Outputs=9
  From11 : From  Commented=on  GotoTag=Tb
  From12 : From  Commented=on  GotoTag=X_hat
  From13 : From  Commented=on  GotoTag=W
  From17 : From  Commented=on  GotoTag=P_
  From18 : From  Commented=on  GotoTag=Fx
  From19 : From  Commented=on  GotoTag=Fx_kalman
  From20 : From  Commented=on  GotoTag=F_hat
  From25 : From  Commented=on  GotoTag=Tb
  From26 : From  Commented=on  GotoTag=X
  From27 : From  Commented=on  GotoTag=W
  From28 : From  Commented=on  GotoTag=P
  From29 : From  Commented=on
  From30 : From  Commented=on  GotoTag=St
  From31 : From  Commented=on  GotoTag=X
  From32 : From  Commented=on  GotoTag=Fx_lr
  From33 : From  Commented=on  GotoTag=Fx
  From34 : From  Commented=on  GotoTag=Fx_rr
  From35 : From  Commented=on  GotoTag=Fx
  From36 : From  Commented=on  GotoTag=Fxf
  From37 : From  Commented=on  GotoTag=Fyr
  From38 : From  Commented=on  GotoTag=Fy
  From39 : From  Commented=on  GotoTag=Fyf
  Gain{2..4,7..8} (5 alike) : Gain  Commented=on  Gain=-1
  Goto12 : Goto  Commented=on  GotoTag=X_hat
  Goto13 : Goto  Commented=on  GotoTag=P_
  Goto14 : Goto  Commented=on  GotoTag=Fx_kalman
  Goto20 : Goto  Commented=on  GotoTag=X
  Goto21 : Goto  Commented=on  GotoTag=P
  Goto22 : Goto  Commented=on  GotoTag=Fx_lr
  Goto23 : Goto  Commented=on  GotoTag=Fx_rr
  Goto24 : Goto  Commented=on  GotoTag=Fxf
  Goto25 : Goto  Commented=on  GotoTag=Fyf
  Goto26 : Goto  Commented=on  GotoTag=Fyr
  MATLAB Function1 : MATLAB Function  Commented=on  TreatAsAtomicUnit=on
  MATLAB Function5 : MATLAB Function  Commented=on  TreatAsAtomicUnit=on
  Scope{12..16} (5 alike) : Scope  Commented=on  NumInputPorts=2
  Scope2 : Scope  Commented=on  NumInputPorts=3
  Sum : Sum  Commented=on  Inputs=|++
  Sum1 : Sum  Commented=on  Inputs=|++
  Sum2 : Sum  Commented=on  Inputs=++|
  Out1 : Outport
  Out2 : Outport  Port=2
  Out3 : Outport  Port=3
  Out4 : Outport  Port=4
  Out5 : Outport  Port=5
  Fx_lr : Outport  Port=6
  Out7 : Outport  Port=7
  Out8 : Outport  Port=8
  Out9 : Outport  Port=9
  Out10 : Outport  Port=10
  Fx_rr : Outport  Port=11
  Out12 : Outport  Port=12
  Out13 : Outport  Port=13
  Out14 : Outport  Port=14
  Out15 : Outport  Port=15
  Out16 : Outport  Port=16
  Out17 : Outport  Port=17
  Out18 : Outport  Port=18
  wires:
  From26/1 -> Delay One Step9/1
  Demux12/7 -> Goto24/1
  Delay One Step4/1 -> MATLAB Function1/4("P ")
  MATLAB Function5/1(X) -> Goto20/1
  Demux2/1 -> Out8/1
  Demux3/1 -> Out15/1
  Demux1/2 -> Scope2/1
  MATLAB Function1/2(P) -> Goto13/1
  From27/1 -> MATLAB Function5/2(w)
  Gain3/1 -> Demux1/1
  Delay One Step3/1 -> MATLAB Function1/1("X ")
  Sum1/1 -> Scope12/1  "Fyf"
  MATLAB Function1/1(X) -> Goto12/1
  From13/1 -> MATLAB Function1/2(w)
  From20/1 -> Gain4/1
  Demux2/3 -> Out12/1
  Demux2/2 -> Scope2/2
  From29/1 -> MATLAB Function5/4(A)
  Delay One Step1/1 -> Gain2/1
  From11/1 -> Delay One Step1/1
  Demux15/3 -> Sum1/2
  Demux13/3 -> Out14/1
  From12/1 -> Delay One Step3/1
  From35/1 -> Gain8/1
  Gain4/1 -> Demux3/1
  Demux13/1 -> Out9/1
  Demux13/2 -> Scope14/1  "Fx_lr"
  From30/1 -> Delay One Step13/1
  From38/1 -> Demux15/1
  Demux12/4 -> Out10/1
  From33/1 -> Gain7/1
  Gain7/1 -> Demux13/1
  From31/1 -> Demux12/1
  Sum/1 -> Scope16/1  "Fxf"
  Delay One Step12/1 -> MATLAB Function5/6("P ")
  Demux13/4 -> Scope15/1  "Fx_rr"
  Demux14/3 -> Sum/2
  MATLAB Function5/2(P) -> Goto21/1
  From32/1 -> Scope14/2  "Fx_lr_hat"
  Demux2/4 -> Out13/1
  From19/1 -> Demux2/1
  From17/1 -> Delay One Step4/1
  Demux12/5 -> Goto22/1
  From37/1 -> Scope13/2  "Fyr_hat"
  Demux14/1 -> Sum/1
  From36/1 -> Scope16/2  "Fxf_hat"
  Demux15/4 -> Sum2/2
  From25/1 -> MATLAB Function5/3(T)
  Demux12/8 -> Goto25/1
  Gain8/1 -> Demux14/1
  MATLAB Function1/3(Fx) -> Goto14/1
  Sum2/1 -> Scope13/1  "Fyr"
  From34/1 -> Scope15/2  "Fx_rr_hat"
  From18/1 -> Gain3/1
  Demux12/1 -> Out4/1
  Demux15/1 -> Sum1/1
  From28/1 -> Delay One Step12/1
  Delay One Step13/1 -> MATLAB Function5/5(St)
  Demux3/3 -> Out17/1
  From39/1 -> Scope12/2  "Fyf_hat"
  Demux3/2 -> Out16/1
  Demux12/9 -> Goto26/1
  Demux15/2 -> Sum2/1
  Delay One Step9/1 -> MATLAB Function5/1("X ")
  Demux12/6 -> Goto23/1
  Demux14/2 -> Fx_lr/1  "Fx_lr"
  Gain2/1 -> MATLAB Function1/3(T)
  Demux14/4 -> Fx_rr/1  "Fx_rr"
  Demux3/4 -> Out18/1
  Demux1/1 -> Out1/1
  Demux1/3 -> Out2/1
  Demux1/4 -> Out3/1
  Demux12/2 -> Out5/1
  In1/1 -> Scope2/3
  Demux12/3 -> Out7/1

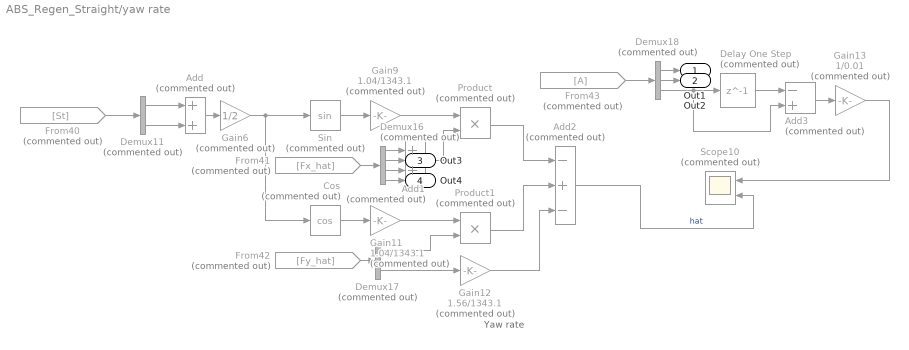
== system ABS_Regen_Straight/yaw rate ==
  note: Yaw rate
  Add : Sum  Commented=on
  Add1 : Sum  Commented=on
  Add2 : Sum  Commented=on  Inputs=-+-
  Add3 : Sum  Commented=on  Inputs=-+
  Cos : Trigonometry  Commented=on  Operator=cos
  Delay One Step : Delay  Commented=on  DelayLength=1
  Demux11 : Demux  Commented=on  Outputs=2
  Demux16 : Demux  Commented=on
  Demux17 : Demux  Commented=on  Outputs=2
  Demux18 : Demux  Commented=on  Outputs=3
  From40 : From  Commented=on  GotoTag=St
  From41 : From  Commented=on  GotoTag=Fx_hat
  From42 : From  Commented=on  GotoTag=Fy_hat
  From43 : From  Commented=on
  Gain11 : Gain  Commented=on  Gain=1.04/1343.1
  Gain12 : Gain  Commented=on  Gain=1.56/1343.1
  Gain13 : Gain  Commented=on  Gain=1/0.01
  Gain6 : Gain  Commented=on  Gain=1/2
  Gain9 : Gain  Commented=on  Gain=1.04/1343.1
  Product : Product  Commented=on
  Product1 : Product  Commented=on
  Scope10 : Scope  Commented=on  NumInputPorts=2
  Sin : Trigonometry  Commented=on
  Out1 : Outport
  Out2 : Outport  Port=2
  Out3 : Outport  Port=3
  Out4 : Outport  Port=4
  wires:
  Gain6/1 -> Cos/1, Sin/1
  Cos/1 -> Gain11/1
  Add1/1 -> Product/2
  Product1/1 -> Add2/2
  Gain9/1 -> Product/1
  Demux16/1 -> Add1/1
  Demux17/1 -> Product1/2
  Demux17/2 -> Gain12/1
  Gain12/1 -> Add2/3
  Add3/1 -> Gain13/1
  Demux18/3 -> Add3/2, Delay One Step/1
  Demux16/2 -> Out3/1
  Gain13/1 -> Scope10/1
  Add2/1 -> Scope10/2  "hat"
  Product/1 -> Add2/1
  Demux18/1 -> Out1/1
  Delay One Step/1 -> Add3/1
  Sin/1 -> Gain9/1
  Demux16/3 -> Add1/2
  From41/1 -> Demux16/1
  Gain11/1 -> Product1/1
  Demux11/1 -> Add/1
  From42/1 -> Demux17/1
  Demux18/2 -> Out2/1
  Demux11/2 -> Add/2
  Demux16/4 -> Out4/1
  Add/1 -> Gain6/1
  From43/1 -> Demux18/1
  From40/1 -> Demux11/1

== matlab function ABS_Regen_Straight/previous KF/MATLAB Function5 ==
  data: X input; w input; T input; A input; St input; X output; P output; P input; Reff data_store_memory; J data_store_memory; Ts data_store_memory; I data_store_memory; M data_store_memory; lf data_store_memory; lr data_store_memory
function [X,P]  = fcn(X,w,T,A,St,P)

global  Reff J Ts I M lf lr;

delta = (St(1)+St(2))/2;

%X = [w_lr w_rr r T F_lr F_rr F_xf F_yf F_yr]
Q = diag([0.000001 0.0001 0.000001 1000 150 150 1000 50000 50000]);

%Z = [w_lr w_rr r T ax ay]
Z = [w(2),w(4),A(3),-T(2),A(1),A(2)]';
R = diag([0.00028 0.00028 0.0000001 0.1 0.001 0.001]);

F = eye(9) + Ts*...
    [0 0 0 -1/J Reff/J 0 0 0 0;
     0 0 0 -1/J 0 Reff/J 0 0 0;
     0 0 0 0 0 0 -lf*sin(delta)/I lf*cos(delta)/I -lr/I;
     zeros(6,9)];

H = [1 0 0 0 0 0 0 0 0;
     0 1 0 0 0 0 0 0 0;
     0 0 1 0 0 0 0 0 0;
     0 0 0 1 0 0 0 0 0;
     0 0 0 0 -1/M -1/M -cos(delta)/M -sin(delta)/M 0;
     0 0 0 0 0 0 -sin(delta)/M cos(delta)/M 1/M];

Xm = F*X;
Pm = F*P*F'+Q;
K = Pm*H'/(H*Pm*H'+R);
X = Xm+K*(Z-H*Xm);
P = (eye(9)-K*H)*Pm;

end

== matlab function ABS_Regen_Straight/MATLAB Function10 ==
  data: ABS input; Tbff input; Pl output; Tbfb input; kappa input; Pr output; Tbf output; Tbr output
function [Pl,Pr,Tbf,Tbr] = fcn(ABS,Tbff,Tbfb,kappa)

if ABS == 1
    Pl = Tbff(1)/(kappa);
    Pr = Tbff(3)/(kappa);
else
    Pl = Tbff(1)/(200);
    Pr = Tbff(3)/(200);
end

Tbf = max(0,min(Tbfb(1),Tbfb(3)));

Tbr = min(Tbff(2)+Tbfb(2),Tbff(4)+Tbfb(4));

== matlab function ABS_Regen_Straight/MATLAB Function2 ==
  data: t input; t output; Ts data_store_memory; ABS input; Tb input; ABS output; Tb output; Fx input; Fxd input; e_ input; e output; Tbr output
function [t,ABS,Tb,e,Tbr]  = fcn(t,ABS,Tb,Fx,Fxd,e_)

Pmax = 5; kpr = 100;

global Ts
t = t + Ts;

%% Error Calculation
e = Fxd-Fx;
edot = e-e_;
%% Torque Controller
Kp = 10; Kd = 10;
if t <= 5
    ABS = 0;
elseif ABS == 1
    Tb_dot = Kp*e + Kd*edot;
    Tb = Tb + Tb_dot;
    ABS = 1;
elseif t <= 5.3 && ABS == 0
    if Fx(2) >= Fxd(2) || Fx(4) >= Fxd(4)
        ABS = 1;
        Tb_dot = Kp*e + Kd*edot;
        Tb = Tb + Tb_dot;
    else
        Tb = Tb + kpr*Pmax/30;
    end
else
    ABS = 0;
end
%%
Tbr = min (Tb(2),Tb(4));

== matlab function ABS_Regen_Straight/MATLAB Function4 ==
  data: t input; Ts data_store_memory; ABS input; Fxd input; Reff data_store_memory; Pl output; Pr output; kappa input; Pl input; Pr input
function [Pl,Pr]  = fcn(t,ABS,Fxd,kappa,Pl,Pr)

Pmax = 5;
global Reff Ts
t = t + Ts;
if t <= 5
    Pl = 0; Pr = 0;
elseif ABS == 1
    %추후에 kpf 대신 kappa 사용
    Pl = 1/kappa*Reff*Fxd(1);    
    Pr = 1/kappa*Reff*Fxd(3);
elseif t <= 5.3 && ABS == 0
    Pl = Pl + Pmax/30;
    Pr = Pr + Pmax/30;
end

== matlab function ABS_Regen_Straight/MATLAB Function5 ==
  data: Fy input; Fxd output; m_s data_store_memory; m_uf data_store_memory; m_ur data_store_memory; lf data_store_memory; lr data_store_memory; h data_store_memory; m_t data_store_memory; D data_store_memory; Fz input; mu input
function Fxd = fcn(Fy,Fz,mu)

Fxd = zeros(4,1);
for i = 1:4
    F = mu^2.*Fz(i)^2-Fy(i)^2;
    if F < 0 
        F = 0;
    end
    Fxd(i) = sqrt(F);
end

== matlab function ABS_Regen_Straight/MATLAB Function6 ==
  data: ABS input; Tb input; Tb output; Fx input; Fxd input; e_ input; e output; Tbf output
function [Tb,e,Tbf]  = fcn(ABS,Tb,Fx,Fxd,e_)

%% Error Calculation
e = Fxd-Fx;
edot = e-e_;

%% Torque Controller
Kp = 0.3; Kd = 1.0;
if ABS == 1
    Tb_dot = Kp*e + Kd*edot;
    Tb = Tb + Tb_dot;
else
    Tb = zeros(4,1);
end

%%
Tbf = min (Tb(1),Tb(3));

== matlab function ABS_Regen_Straight/MATLAB Function7 ==
  data: Tf_regen input; Tr_regen input; P_input output; Pl input; Pr input
function P_input  = fcn(Tf_regen,Tr_regen,Pl,Pr)

%% Pressure-Torque Gain
Kf = 150; Kr = 100;

%% Control Input
LF = Pl + Tf_regen/Kf;
LR = Tr_regen/Kr;
RF = Pr + Tf_regen/Kf;
RR = Tr_regen/Kr;

P_input = [LF LR RF RR]';

== matlab function ABS_Regen_Straight/MATLAB Function8 ==
  data: t output; t input; ABS input; Ts data_store_memory; Tb input; Tb output; ABS output; Fx input; Fxd input; Reff data_store_memory
function [t,Tb,ABS]   = fcn(t,ABS,Tb,Fx,Fxd)

Pmax = 5; kpr = 100; kpf = 200; ts = 0.3;

global Ts Reff
t = t + Ts;

%% Torque Controller
if t <= 5
    ABS = 0;
elseif ABS == 1
    Tb = Fxd*Reff;
elseif t <= (5+ts) && ABS == 0
    if Fx(2) >= Fxd(2) || Fx(4) >= Fxd(4)
        ABS = 1;
        Tb = Fxd*Reff;
    else
        Tb([2,4]) = Tb([2,4]) + kpr*Pmax/ts*Ts;
        Tb([1,3]) = Tb([1,3]) + kpf*Pmax/ts*Ts;
    end
else
    if Fx(2) >= Fxd(2) || Fx(4) >= Fxd(4)
        ABS = 1;
    else
        ABS = 0;
    end
end

== matlab function ABS_Regen_Straight/MATLAB Function9 ==
  data: ABS input; Tb input; Fx input; Fxd input; e_ input; Ts data_store_memory; Tb output; e output; Reff data_store_memory
function [Tb,e]   = fcn(ABS,Tb,Fx,Fxd,e_)

kpr = 100; kpf = 150;

global Ts Reff

e = Fx-Fxd;
edot = e-e_;

%% Torque Controller
Kpf = 0.03; Kdf = 0.11;
Kpr = 0.005; Kdr = 0.4;
% Kpf = 0.02; Kdf = 0.11;
% Kpr = 0.004; Kdr = 0.3;
if ABS == 1
    Tbdotf = Kpf*e + Kdf*edot;
    Tbdotr = Kpr*e + Kdr*edot;
    Tb([1,3]) = Tb([1,3]) - Tbdotf([1,3]);
    Tb([2,4]) = Tb([2,4]) - Tbdotr([2,4]);
else
    Tb = zeros(4,1);
end

== matlab function ABS_Regen_Straight/MATLAB Function11 ==
  data: w input; kappa output; w_ input; Fxhat input; Reff data_store_memory; Pc input; J data_store_memory
function kappa = fcn(w,w_,Fxhat,Pc)

global Reff J

wdot = w-w_;

kappa = (Reff*(Fxhat(1)+Fxhat(3))-J*(wdot(1)+wdot(3)))/(Pc(1)+Pc(2));

== matlab function ABS_Regen_Straight/MATLAB Function12 ==
  data: Fz input; Fyhat output; Fy input
function Fyhat = fcn(Fz, Fy)

kf = Fz(1)/Fz(3);
kr = Fz(2)/Fz(4);

Fylf = kf/(1+kf)*Fy(1);
Fyrf = 1/(1+kf)*Fy(1);
Fylr = kr/(1+kr)*Fy(2);
Fyrr = 1/(1+kf)*Fy(2);

Fyhat = [Fylf Fylr Fyrf Fyrr]';

== matlab function ABS_Regen_Straight/previous KF/MATLAB Function1 ==
  data: X input; w input; T input; X output; P output; P input; Fx output; Reff data_store_memory; J data_store_memory; Ts data_store_memory
function [X,P,Fx]  = fcn(X,w,T,P)

global  Reff J Ts;

Qlf = [1 0;0 500000]; Qlr = [0.01 0;0 900]; Qrf = [1 0;0 500000]; Qrr = [1 0;0 500000]; Q = [Qlf Qlr Qrf Qrr];
Rlf = 1; Rlr = 0.01; Rrf = 1; Rrr = 1; R = [Rlf Rlr Rrf Rrr];

F = [1 Reff/J*Ts;0 1]; G = [-1/J*Ts;0]; H = [1 0];

for i = 1:4
    xm = F*X(:,i)+G*T(i);
    Pm = F*P(:,2*i-1:2*i)*F'+Q(:,2*i-1:2*i);
    K = Pm*H'/(H*Pm*H'+R(i));
    X(:,i) = xm+K*(w(i)-H*xm);
    P(:,2*i-1:2*i) = (eye(2)-K*H)*Pm;
end
Fx = X(2,:);

== matlab function ABS_Regen_Straight/MATLAB Function ==
  data: A input; Fz output; m_s data_store_memory; m_uf data_store_memory; m_ur data_store_memory; lf data_store_memory; lr data_store_memory; h data_store_memory; m_t data_store_memory; D data_store_memory
function Fz = fcn(A)

a = [9.8 A(1) A(2)]';

global m_s m_uf m_ur lf lr h m_t D

L = lf+lr;
Mz = [lr/(2*L)*m_s+1/2*m_uf+m_t -h/(2*L)*m_s -h/(2*D)*m_s;
     lf/(2*L)*m_s+1/2*m_ur+m_t h/(2*L)*m_s -h/(2*D)*m_s;
     lr/(2*L)*m_s+1/2*m_uf+m_t -h/(2*L)*m_s h/(2*D)*m_s;
     lf/(2*L)*m_s+1/2*m_ur+m_t h/(2*L)*m_s h/(2*D)*m_s];

Fz = Mz*a;

== matlab function ABS_Regen_Straight/MATLAB Function3 ==
  data: X input; w input; Pc input; T input; A input; St_ input; St input; X output; P output; P input; Reff data_store_memory; J data_store_memory; Ts data_store_memory; I data_store_memory; M data_store_memory; lf data_store_memory; lr data_store_memory; D data_store_memory
function [X,P]  = fcn(X,w,Pc,T,A,St_,St,P)

global  Reff J Ts I M lf lr D;
T(1) = 0;
delta_ = (St_(1)+St_(2))/2;
delta = (St(1)+St(2))/2;

%X = [w_lf w_lr w_rf w_rr k Pl Pr r Tf Tr F_lf F_lr F_rf F_rr F_yf F_yr]
Q = diag([0.00001 0.00001 0.00001 0.00001 0.001 100 100 0.000001 1000 1000 100 100 100 100 1000 1000]);

%Z = [w_lf w_lr w_rf w_rr Pl Pr r Tf Tr ax ay]
Z = [w(1),w(2),w(3),w(4),Pc(1),Pc(2),A(3),-T(1),-T(2),A(1),A(2)]';
R = diag([0.00028 0.00028 0.00028 0.00028 0.001 0.001 0.0000001 0.001 0.001 0.0001 0.0001]);

F = eye(16) + Ts*...
    [0 0 0 0 -1/J*X(6) -1/J*X(5) 0 0 -1/J 0 Reff/J 0 0 0 0 0;
     0 0 0 0 0 0 0 0 0 -1/J 0 Reff/J 0 0 0 0;
     0 0 0 0 -1/J*X(7) 0 -1/J*X(5) 0 -1/J 0 0 0 Reff/J 0 0 0;
     0 0 0 0 0 0 0 0 0 -1/J 0 0 0 Reff/J 0 0;
     zeros(3,16);
     0 0 0 0 0 0 0 0 0 0 D/2/I*cos(St_(1))-lf/I*sin(St_(1)) D/2/I -D/2/I*cos(St_(2))-lf/I*sin(St_(2)) -D/2/I lf/I*cos(delta_) -lr/I;
     zeros(8,16)];

H = [1 0 0 0 0 0 0 0 0 0 0 0 0 0 0 0;
     0 1 0 0 0 0 0 0 0 0 0 0 0 0 0 0;
     0 0 1 0 0 0 0 0 0 0 0 0 0 0 0 0;
     0 0 0 1 0 0 0 0 0 0 0 0 0 0 0 0;
     0 0 0 0 0 1 0 0 0 0 0 0 0 0 0 0;
     0 0 0 0 0 0 1 0 0 0 0 0 0 0 0 0;
     0 0 0 0 0 0 0 1 0 0 0 0 0 0 0 0;
     0 0 0 0 0 0 0 0 1 0 0 0 0 0 0 0;
     0 0 0 0 0 0 0 0 0 1 0 0 0 0 0 0;
     0 0 0 0 0 0 0 0 0 0 -cos(St(1))/M -1/M -cos(St(2))/M -1/M -sin(delta)/M 0;
     0 0 0 0 0 0 0 0 0 0 -sin(St(1))/M 0 -sin(St(2))/M 0 cos(delta)/M 1/M];

X(1) = X(1) + (Reff/J*X(11)-1/J*(X(5)*X(6)+X(9)))*Ts;
X(2) = X(2) + (Reff/J*X(12)-1/J*X(10))*Ts;
X(3) = X(3) + (Reff/J*X(13)-1/J*(X(5)*X(7)+X(9)))*Ts;
X(4) = X(4) + (Reff/J*X(14)-1/J*X(10))*Ts;
X(8) = X(8) + ((D/2/I*cos(St_(1))-lf/I*sin(St_(1)))*X(11)+D/2/I*X(12)+(-D/2/I*cos(St_(2))-lf/I*sin(St_(2)))*X(13)-D/2/I*X(14)+lf/I*cos(delta_)*X(15)-lr/I*X(16))*Ts;



Xm = X;
Pm = F*P*F'+Q;
K = Pm*H'/(H*Pm*H'+R);
X = Xm+K*(Z-H*Xm);
P = (eye(16)-K*H)*Pm;

end

== matlab function ABS_Regen_Straight/MATLAB Function1 ==
  data: Fy input; Fxd output; m_s data_store_memory; m_uf data_store_memory; m_ur data_store_memory; lf data_store_memory; lr data_store_memory; h data_store_memory; m_t data_store_memory; D data_store_memory; Fz input
function Fxd = fcn(Fy,Fz)

mu = 0.5;

Fxd = zeros(4,1);
for i = 1:4
    F = mu^2.*Fz(i)^2-Fy(i)^2;
    if F < 0 
        F = 0;
    end
    Fxd(i) = sqrt(F);
end
